simulink model "Untitled1"  (R2016b)
settings: Solver=VariableStepAuto  StartTime=0.0  StopTime=10.0  RelTol=1e-3
settings Model: Creator=Yasna  LastModifiedBy=Yasna

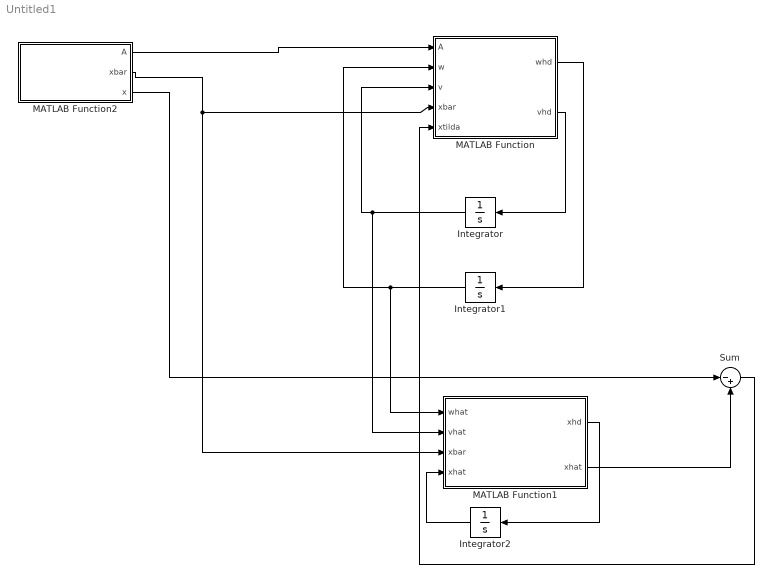
== system Untitled1 ==
  Integrator : Integrator
  Integrator1 : Integrator
  Integrator2 : Integrator
  MATLAB Function : MATLAB Function  TreatAsAtomicUnit=on
  MATLAB Function1 : MATLAB Function  TreatAsAtomicUnit=on
  MATLAB Function2 : MATLAB Function  TreatAsAtomicUnit=on
  Sum : Sum  Inputs=|-+
  wires:
  MATLAB Function/1(whd) -> Integrator1/1
  MATLAB Function/2(vhd) -> Integrator/1
  Integrator1/1 -> MATLAB Function1/1(what), MATLAB Function/2(w)
  Integrator/1 -> MATLAB Function1/2(vhat), MATLAB Function/3(v)
  MATLAB Function2/1(A) -> MATLAB Function/1(A)
  MATLAB Function2/2(xbar) -> MATLAB Function1/3(xbar), MATLAB Function/4(xbar)
  MATLAB Function1/1(xhd) -> Integrator2/1
  Integrator2/1 -> MATLAB Function1/4("xhat ")
  MATLAB Function2/3(x) -> Sum/1
  MATLAB Function1/2(xhat) -> Sum/2
  Sum/1 -> MATLAB Function/5(xtilda)

== matlab function Untitled1/MATLAB Function2 ==
  data: A output; xbar output; x output
function [A,xbar,x]= fcn
n=4;
A=-eye(n);
xbar=
x=

== matlab function Untitled1/MATLAB Function ==
  data: A input; whd output; w input; v input; xbar input; vhd output; xtilda input
function [whd,vhd]= fcn(A,w,v,xbar,xtilda)
eta1 = 0.1;
eta2 = 0.1;
ro1 = 0.5;
ro2 = 0.5;
whd=-eta1*xtilda

== matlab function Untitled1/MATLAB Function1 ==
  data: what input; vhat input; xbar input; xhat input; xhd output; xhat output
function [xhd,xhat]= fcn(what,vhat,xbar,xhat)
sig=zeros(4,1);
for i=0:4
    sig[i] = 2/(1 + exp(-2*vhat(i,1)*xbar)) - 1
    
ghat=what*sig;
xhd=ghat+A*xhat;
